simulink model "Interp"  (Simulink 8.9)
settings: Solver=ode45  StartTime=0.0  StopTime=60.0  MaxStep=.05  RelTol=1e-3  AbsTol=1e-6
undefined symbols (not defined in the file or in its folder): a, b, c, d
settings Model: SuppressorTable=22 serialization::archive 11 0 6 0 0 0 11 0  Creator=vise  LastModifiedBy=dangd  ExtModeTrigMode=oneshot  ExtModeArmWhenConnect=off  ExtModeAutoUpdateStatusClock=off
settings DataIOCC: LimitDataPoints=off
settings OptimizationCC: BooleanDataType=off  ExpressionDepthLimit=2147483647  InitFltsAndDblsToZero=on
settings DebuggingCC: SaveWithParameterizedLinksMsg=none  SignalResolutionControl=TryResolveAllWithWarning  MultiTaskDSMMsg=warning  MultiTaskCondExecSysMsg=none
settings HardwareCC: TargetUnknown=on
settings RTWCC: TemplateMakefile=grt_unix.tmf
settings GRTTargetCC: GeneratePreprocessorConditionals=Use local settings

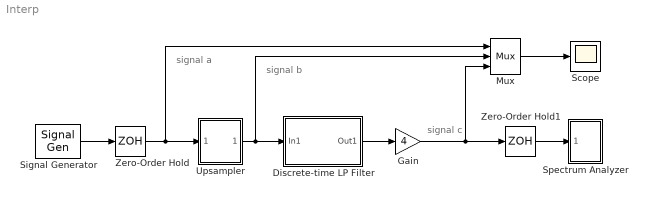
== system Interp ==
  note: signal c
  note: signal b
  note: signal a
  Discrete-time LP Filter : Subsystem  mask(butter){MaskParam1=pi/4, MaskParam2=10, MaskParam3=0.25}
      mask prompts: MaskParam1 "Cutoff frequency (0 to pi):"; MaskParam2 "Order:"; MaskParam3 "Sample time:"
      mask help:
      | Butterworth low pass filter.
      | (Requires Signal Processing Toolbox)
      mask init:
      | [a,b,c,d]=butter(MaskParam2,MaskParam1/pi); ts=MaskParam3; [num,den]=ss2tf(a,b,c,d,1); if (MaskParam2 <= 8), [a,b,c,d]=tf2ss(num,den); end; h=freqz(num,den,64);
      mask Help: IIR Butterworth low pass filter using MATLAB's butter command.
      mask Display: plot(1:64,abs(h))
  Gain : Gain  Gain=4  SaturateOnIntegerOverflow=on  OutDataTypeStr=Inherit: Same as input  ParamDataTypeStr=Inherit: Same as input
  Mux : Mux  Inputs=3
  Scope : Scope
  Signal Generator : SignalGenerator  Amplitude=1.000000  Frequency=0.1
  Spectrum Analyzer : Subsystem  mask(Spectrum analyzer.){N=1024, T_s=.05, plot_period=10}
      mask prompts: N "Number of sample points:"; T_s "Sampling period (sec):"; plot_period "Plotting Period (sec):"
      mask Help: EE438 Lab utility; See Prof. Bouman.
      mask Display: plot(0,0,100,100,[14,91,91,14,14],[86,86,40,40,86],[85,82,80,79,75,67,63,60,57,53,41,36,33,27,24],[49,50,53,50,49,51,54,66,54,50,50,52,81,51,49])
  Upsampler : Subsystem  mask(D-T interpolator){T=1, L=4}
      mask prompts: T "Input sampling period:"; L "Upsampling factor:"
      mask Display: disp('L')
  Zero-Order Hold : ZeroOrderHold
  Zero-Order Hold1 : ZeroOrderHold  SampleTime=.05
  wires:
  Zero-Order Hold1/1 -> Spectrum Analyzer/1(input signal)
  Mux/1 -> Scope/1
  Gain/1 -> Zero-Order Hold1/1, Mux/3
  Discrete-time LP Filter/1(Out1) -> Gain/1
  Zero-Order Hold/1 -> Mux/1, Upsampler/1(in_1)
  Upsampler/1(out_1) -> Discrete-time LP Filter/1(In1), Mux/2
  Signal Generator/1 -> Zero-Order Hold/1

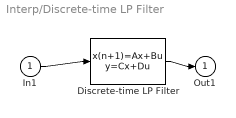
== system Interp/Discrete-time LP Filter ==
  In1 : Inport
  Discrete-time LP Filter : DiscreteStateSpace  A=a  B=b  C=c  D=d  SampleTime=ts
  Out1 : Outport
  wires:
  In1/1 -> Discrete-time LP Filter/1
  Discrete-time LP Filter/1 -> Out1/1

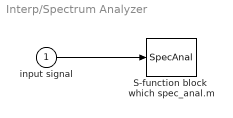
== system Interp/Spectrum Analyzer ==
  input signal : Inport
  S-function block  which spec_anal.m : S-Function  FunctionName=SpecAnal  Parameters=N,T_s,plot_period  SFunctionDeploymentMode=off  EnableBusSupport=off
  wires:
  input signal/1 -> S-function block  which spec_anal.m/1

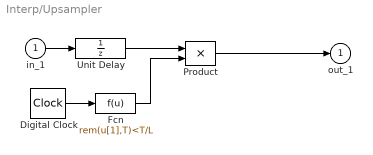
== system Interp/Upsampler ==
  in_1 : Inport
  Digital Clock : DigitalClock  SampleTime=T/L
  Fcn : Fcn  Expr=rem(u[1],T)<T/L
  Product : Product  SaturateOnIntegerOverflow=on  RndMeth=Zero  InputSameDT=on  OutDataTypeStr=Inherit: Same as first input
  Unit Delay : UnitDelay  SampleTime=T/L
  out_1 : Outport  InitialOutput=0
  wires:
  Product/1 -> out_1/1
  Fcn/1 -> Product/2
  Unit Delay/1 -> Product/1
  in_1/1 -> Unit Delay/1
  Digital Clock/1 -> Fcn/1
